simulink subsystem "bh_COMPONENT_model_7dof_car_SCAPE_activeSUSP"  (R2021a)
settings: Solver=VariableStepAuto  StartTime=0.0  StopTime=10.0  RelTol=1e-3
model mask{L_b=0, L_f=0, L_R=0, L_L=0, m_c=0, I_cZ=0, I_cX=0, m_bR=0, m_fR=0, m_bL=0, m_fL=0, k_bR=0, k_fR=0, k_bL=0, k_fL=0, k_bRG=0, k_fRG=0, k_bLG=0, k_fLG=0, c_bR=0, c_fR=0, c_bL=0, c_fL=0, c_bRG=0, c_fRG=0, c_bLG=0, c_fLG=0, IC_pos=zeros(7,1), IC_vel=zeros(7,1)}
  mask prompts: L_b "L_b   (m)"; L_f "L_f   (m)"; L_R "L_R   (m)"; L_L "L_L   (m)"; m_c "m_c     (kg)"; I_cZ "I_cZ      (kg.m^2)"; I_cX "I_cX      (kg.m2)"; m_bR "m_bR   (kg)"; m_fR "m_fR    (kg)"; m_bL "m_bL   (kg)"; m_fL "m_fL    (kg)"; k_bR "k_bR   (N/m)"; k_fR "k_fR   (N/m)"; k_bL "k_bL   (N/m)"; k_fL "k_fL    (N/m)"; k_bRG "k_bRG   (N/m)"; k_fRG "k_fRG   (N/m)"; k_bLG "k_bLG   (N/m)"; k_fLG "k_fLG    (N/m)"; c_bR "c_bR  (N.s/m)"; c_fR "c_fR  (N.s/m)"; c_bL "c_bL  (N.s/m)"; c_fL "c_fL  (N.s/m)"; c_bRG "c_bRG  (N.s/m)"; c_fRG "c_fRG  (N.s/m)"; c_bLG "c_bLG  (N.s/m)"; c_fLG "c_fLG  (N.s/m)"
undefined symbols (not defined in the file): X, Y, Z
libraries: sm_lib x44, fl_lib x36, nesl_utility x18
(part 2 of 2)

== system bh_COMPONENT_model_7dof_car_SCAPE_activeSUSP/CAR_BODY/CAR_SYS/Subsystem ==
  " CAR" : sm_lib/Body Elements/Brick Solid  GraphicAmbientColor=[0.15 0.15 0.15 1.0]  BasedOnType=Density  BrickDimensions=[(L_b+L_f), 0.25, (L_R+L_L)]  BrickDimensionUnits=m  CenterOfMass=G_rel_to_R  CenterOfMassUnits=m  GraphicDiffuseColor=[0.0 1.0 0.2]  Density=1000  DensityUnits=kg/m^3  DoExposeReferenceFrame=on  GraphicEmissiveColor=[0.0 0.0 0.0 1.0]  ExportEntireGeometry=off  SerializedFrames=<Frames><Frame><Id>Frame1</Id><Value><Name>A</Name><Origin><Source>GeometricFeature</Source><FeatureName>+z -x curve</FeatureName></Origin><PrimaryAxis><DefinedDirection>+Z</DefinedDirection><Source>ReferenceFrame</Source><SourceDirection>+Z</SourceDirection><FeatureName></FeatureName></PrimaryAxis><SecondaryAxis><DefinedDirection>+X</DefinedDirection><Source>ReferenceFrame</Source><SourceDirection>+X</SourceDirection><FeatureName></FeatureName></SecondaryAxis></Value></Frame><Frame><Id>Frame2</Id><Value><Name>B</Name><Origin><Source>GeometricFeature</Source><FeatureName>+z +x curve</FeatureName></Origin><PrimaryAxis><DefinedDirection>+Z</DefinedDirection><Source>ReferenceFrame</Source><SourceDirection>+Z</SourceDirection><FeatureName></FeatureName></PrimaryAxis><SecondaryAxis><DefinedDirection>+X</DefinedDirection><Source>ReferenceFrame</Source><SourceDirection>+X</SourceDirection><FeatureName></FeatureName></SecondaryAxis></Value></Frame><Frame><Id>Frame3</Id><Value><Name>C</Name><Origin><Source>GeometricFeature</Source><FeatureName>-z +x curve</FeatureName></Origin><PrimaryAxis><DefinedDirection>+Z</DefinedDirection><Source>ReferenceFrame</Source><SourceDirection>+Z</SourceDirection><FeatureName></FeatureName></PrimaryAxis><SecondaryAxis><DefinedDirection>+X</DefinedDirection><Source>ReferenceFrame</Source><SourceDirection>+X</SourceDirection><FeatureName></FeatureName></SecondaryAxis></Value></Frame><Frame><Id>Frame4</Id><Value><Name>D</Name><Origin><Source>GeometricFeature</Source><FeatureName>-z -x curve</FeatureName></Origin><PrimaryAxis><DefinedDirection>+Z</DefinedDirection><Source>ReferenceFrame</Source><SourceDirection>+Z</SourceDirection><FeatureName></FeatureName></PrimaryAxis><SecondaryAxis><DefinedDirection>+X</DefinedDirection><Source>ReferenceFrame</Source><SourceDirection>+X</SourceDirection><FeatureName></FeatureName></SecondaryAxis></Value></Frame><Frame><Id>Frame5</Id><Value><Name>CoM</Name><Origin><Source>CenterOfMassFrame</Source><FeatureName></FeatureName></Origin><PrimaryAxis><DefinedDirection>+Z</DefinedDirection><Source>ReferenceFrame</Source><SourceDirection>+Z</SourceDirection><FeatureName></FeatureName></PrimaryAxis><SecondaryAxis><DefinedDirection>+X</DefinedDirection><Source>ReferenceFrame</Source><SourceDirection>+X</SourceDirection><FeatureName></FeatureName></SecondaryAxis></Value></Frame></Frames>  MarkerShape=Sphere  MarkerSize=10  GraphicType=FromGeometry  InertiaType=Custom  Mass=m  MassUnits=kg  MomentsOfInertia="[I_X ,  5*I_X ,  I_Z]"  MomentsOfInertiaUnits=kg*m^2  GraphicOpacity=1.0  ProductsOfInertia=[0 0 0]  ProductsOfInertiaUnits=kg*m^2  GraphicShininess=75  GraphicSpecularColor=[0.5 0.5 0.5 1.0]  GraphicVisPropType=SimpleVisualProperties
  R : sm_lib/Body Elements/Graphic  Commented=on  GraphicType=Marker  MarkerShape=Frame  MarkerSize=30  GraphicVisPropType=SimpleVisualProperties  GraphicDiffuseColor=[0.0 0.2 1.0]  GraphicSpecularColor=[0.5 0.5 0.5 1.0]  GraphicAmbientColor=[0.15 0.15 0.15 1.0]  GraphicEmissiveColor=[0.0 0.0 0.0 1.0]  GraphicShininess=75  GraphicOpacity=1.0
  A : PMIOPort  Side=Left
  B : PMIOPort  Port=2  Side=Left
  C : PMIOPort  Port=3  Side=Left
  D : PMIOPort  Port=4  Side=Left
  COM : PMIOPort  Port=5  Side=Right
  connections:
  R/RConn1 -- " CAR"/RConn1
  " CAR"/LConn1 -- A/RConn1
  " CAR"/LConn3 -- D/RConn1
  " CAR"/RConn3 -- COM/RConn1
  " CAR"/RConn2 -- C/RConn1
  " CAR"/LConn2 -- B/RConn1

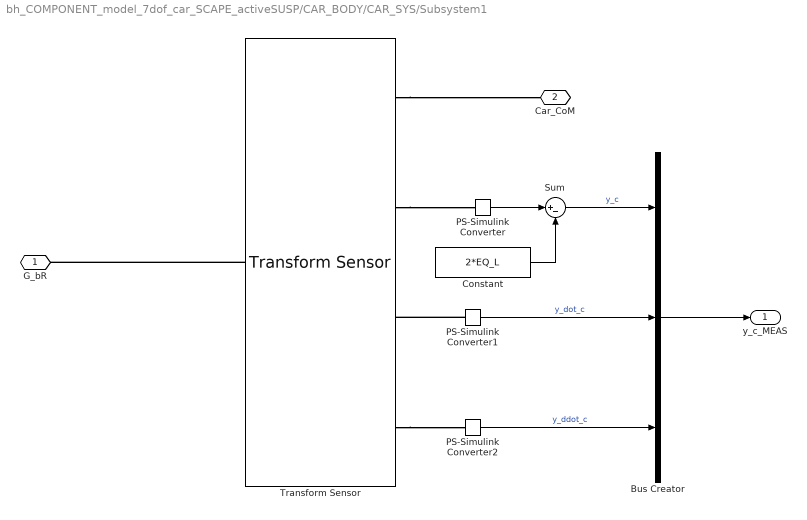
== system bh_COMPONENT_model_7dof_car_SCAPE_activeSUSP/CAR_BODY/CAR_SYS/Subsystem1 ==
  Bus Creator : BusCreator  Inputs=3
  Constant : Constant  Value=2*EQ_L
  PS-Simulink Converter : nesl_utility/PS-Simulink Converter  PhysicalDomain=network_engine_domain  SubClassName=ps_output  LeftPortType=input  RightPortType=output  PseudoPeriodic=off  Frequencies=[]  Unit=m  AffineConversion=off
      settings: SourceProductBaseCode=PW,SS
  PS-Simulink Converter1 : nesl_utility/PS-Simulink Converter  PhysicalDomain=network_engine_domain  SubClassName=ps_output  LeftPortType=input  RightPortType=output  PseudoPeriodic=off  Frequencies=[]  Unit=m/s  AffineConversion=off
      settings: SourceProductBaseCode=PW,SS
  PS-Simulink Converter2 : nesl_utility/PS-Simulink Converter  PhysicalDomain=network_engine_domain  SubClassName=ps_output  LeftPortType=input  RightPortType=output  PseudoPeriodic=off  Frequencies=[]  Unit=m/s^2  AffineConversion=off
      settings: SourceProductBaseCode=PW,SS
  Sum : Sum  Inputs=|+-
  Transform Sensor : sm_lib/Frames and Transforms/Transform Sensor  MeasurementFrame=World  SenseAngle=off  SenseAxis=off  SenseAngle1=off  SenseAngle2=off  SenseAngle3=off  SenseQ=off  SenseR=off  SenseOmegaX=off  SenseOmegaY=off  SenseOmegaZ=off  SenseOmega1=off  SenseOmega2=off  SenseOmega3=off  SenseQDot=off  SenseRDot=off  SenseAlphaX=off  SenseAlphaY=off  SenseAlphaZ=off  SenseAlpha1=off  SenseAlpha2=off  SenseAlpha3=off  SenseQDDot=off  SenseRDDot=off  SenseX=off  SenseY=on  SenseZ=off  SenseRad=off  SenseAzim=off  SenseDist=off  SenseInc=off  SenseXDot=off  SenseYDot=on  SenseZDot=off  SenseRadDot=off  SenseAzimDot=off  SenseDistDot=off  SenseIncDot=off  SenseXDDot=off  SenseYDDot=on  SenseZDDot=off  SenseRadDDot=off  SenseAzimDDot=off  SenseDistDDot=off  SenseIncDDot=off
  G_bR : PMIOPort  Side=Left
  Car_CoM : PMIOPort  Port=2  Side=Right
  y_c_MEAS : Outport
  wires:
  Bus Creator/1 -> y_c_MEAS/1
  PS-Simulink Converter2/1 -> Bus Creator/3  "y_ddot_c"
  PS-Simulink Converter1/1 -> Bus Creator/2  "y_dot_c"
  Sum/1 -> Bus Creator/1  "y_c"
  Constant/1 -> Sum/2
  PS-Simulink Converter/1 -> Sum/1
  connections:
  Transform Sensor/RConn4 -- PS-Simulink Converter2/LConn1
  PS-Simulink Converter1/LConn1 -- Transform Sensor/RConn3
  Transform Sensor/RConn2 -- PS-Simulink Converter/LConn1
  Transform Sensor/LConn1 -- G_bR/RConn1
  Transform Sensor/RConn1 -- Car_CoM/RConn1

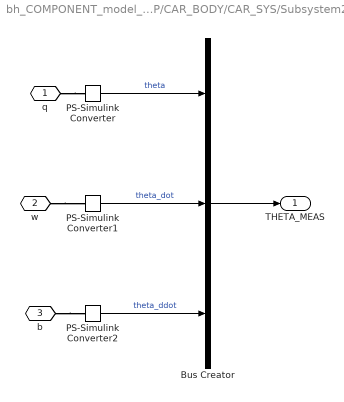
== system bh_COMPONENT_model_7dof_car_SCAPE_activeSUSP/CAR_BODY/CAR_SYS/Subsystem2 ==
  Bus Creator : BusCreator  Inputs=3
  PS-Simulink Converter : nesl_utility/PS-Simulink Converter  PhysicalDomain=network_engine_domain  SubClassName=ps_output  LeftPortType=input  RightPortType=output  PseudoPeriodic=off  Frequencies=[]  Unit=rad  AffineConversion=off
      settings: SourceProductBaseCode=PW,SS
  PS-Simulink Converter1 : nesl_utility/PS-Simulink Converter  PhysicalDomain=network_engine_domain  SubClassName=ps_output  LeftPortType=input  RightPortType=output  PseudoPeriodic=off  Frequencies=[]  Unit=rad/s  AffineConversion=off
      settings: SourceProductBaseCode=PW,SS
  PS-Simulink Converter2 : nesl_utility/PS-Simulink Converter  PhysicalDomain=network_engine_domain  SubClassName=ps_output  LeftPortType=input  RightPortType=output  PseudoPeriodic=off  Frequencies=[]  Unit=rad/s^2  AffineConversion=off
      settings: SourceProductBaseCode=PW,SS
  q : PMIOPort  Side=Left
  w : PMIOPort  Port=2  Side=Left
  b : PMIOPort  Port=3  Side=Left
  THETA_MEAS : Outport
  wires:
  PS-Simulink Converter2/1 -> Bus Creator/3  "theta_ddot"
  PS-Simulink Converter1/1 -> Bus Creator/2  "theta_dot"
  Bus Creator/1 -> THETA_MEAS/1
  PS-Simulink Converter/1 -> Bus Creator/1  "theta"
  connections:
  b/RConn1 -- PS-Simulink Converter2/LConn1
  w/RConn1 -- PS-Simulink Converter1/LConn1
  q/RConn1 -- PS-Simulink Converter/LConn1

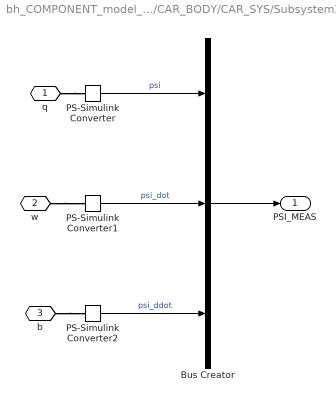
== system bh_COMPONENT_model_7dof_car_SCAPE_activeSUSP/CAR_BODY/CAR_SYS/Subsystem3 ==
  Bus Creator : BusCreator  Inputs=3
  PS-Simulink Converter : nesl_utility/PS-Simulink Converter  PhysicalDomain=network_engine_domain  SubClassName=ps_output  LeftPortType=input  RightPortType=output  PseudoPeriodic=off  Frequencies=[]  Unit=rad  AffineConversion=off
      settings: SourceProductBaseCode=PW,SS
  PS-Simulink Converter1 : nesl_utility/PS-Simulink Converter  PhysicalDomain=network_engine_domain  SubClassName=ps_output  LeftPortType=input  RightPortType=output  PseudoPeriodic=off  Frequencies=[]  Unit=rad/s  AffineConversion=off
      settings: SourceProductBaseCode=PW,SS
  PS-Simulink Converter2 : nesl_utility/PS-Simulink Converter  PhysicalDomain=network_engine_domain  SubClassName=ps_output  LeftPortType=input  RightPortType=output  PseudoPeriodic=off  Frequencies=[]  Unit=rad/s^2  AffineConversion=off
      settings: SourceProductBaseCode=PW,SS
  q : PMIOPort  Side=Left
  w : PMIOPort  Port=2  Side=Left
  b : PMIOPort  Port=3  Side=Left
  PSI_MEAS : Outport
  wires:
  PS-Simulink Converter2/1 -> Bus Creator/3  "psi_ddot"
  PS-Simulink Converter1/1 -> Bus Creator/2  "psi_dot"
  Bus Creator/1 -> PSI_MEAS/1
  PS-Simulink Converter/1 -> Bus Creator/1  "psi"
  connections:
  b/RConn1 -- PS-Simulink Converter2/LConn1
  w/RConn1 -- PS-Simulink Converter1/LConn1
  q/RConn1 -- PS-Simulink Converter/LConn1
